simulink model "IP_nonLinearSys_Openloop_KF"  (R2015a)
settings: Solver=ode5  StartTime=0.0  StopTime=30  FixedStep=0.01  RelTol=1e-3
undefined symbols (not defined in the file): A, B, C, Continuous, D, sigbuilder_block, Time, Ts
libraries: ctrlSharedLib x1
settings Model: Creator=Fares  LastModifiedBy=Fares

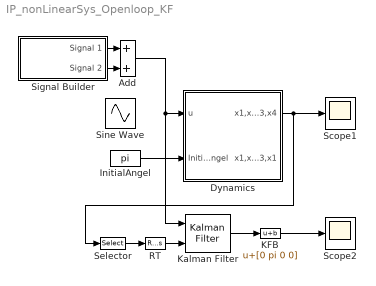
== system IP_nonLinearSys_Openloop_KF ==
  Add : Sum
  Dynamics : Subsystem  mask{mc=1.12, mpw=0.095, mps=0.025, M=9.4, fp=0.000107443, J=0.013935418, l=0.033245968, g=9.81}
      mask prompts: mc "Cart mass [kg]"; mpw "Pendulum weight mass [kg]"; mps "Pendulum stick mass [kg]"; M "Maximum control [N]"; fp "Pendulum friction [kg*m2/s]"; J "Moment of inertia [kg*m2]"; l "Distance: axis of rotation-mass center [m]"; g "Gravetational acceleration [m/s2]"
      mask init:
      | mp = mpw + mps;
      | a = l^2 + J/(mc + mp);
      | mi = (mc + mp)*l;
      mask Display: plot([0],[-2.5],[5],[4.5],[0 5],[0 0],[0 5],[0.1 0.1],[0 2],[1 1],[2.5 5],[1 1],[2 2.5 2.5 2 2],[1.25 1.25 0.75 0.75 1.25],[2.25 1.5],[1 -2.5]);
  InitialAngel : Constant  Value=pi
  KFB : Bias  Bias=[0 pi 0 0]
  Kalman Filter : ctrlSharedLib/Kalman Filter  TimeDomain=Continuous-Time  UseCurrentEstimator=on  ModelSource=Individual A, B, C, D matrices  ModelSourceVariable=ss(A,B,C,D,Ts)  A=A  B=B  C=C  D=D  NumberOfStates=1  NumberOfInputs=1  NumberOfOutputs=1  InitialEstimateSource=Dialog  X0=[0; 0; 0; 0]  P0=10  UseK=off  UseGH=off  NumberOfProcessNoiseInputs=1  G=1  TimeInvariantG=on  H=0  TimeInvariantH=on  Q=diag([1 1 500 8000])  TimeInvariantQ=on  R=diag([1e-03 0.1])  TimeInvariantR=on  N=0  TimeInvariantN=on  AddInputPort=on  AddEnablePort=off  ExternalReset=none  OutputEstimatedY=off  OutputP=off  Ts=-1
  RT : RateTransition
  Scope1 : Scope
      settings: ShowLegends=on
  Scope2 : Scope
      settings: ShowLegends=on
  Selector : Selector  InputPortWidth=4  Indices=[1 3]
  Signal Builder : Subsystem  Tag=STV Subsys  LoadFcn=sigbuilder_block('load');  StartFcn=sigbuilder_block('start');  StopFcn=sigbuilder_block('stop');  ClipboardFcn=sigbuilder_block('clipboard');  mask(Sigbuilder block){}
      mask help: Simulink:masks:SigbuilderBlock_MD
      mask init:
      | if ~strcmp(get_param(bdroot(gcbh),'SimulationStatus'),'stopped') tuvar = sigbuilder_block('maskInit'); end
      settings: CopyFcn=sigbuilder_block('copy');  DeleteFcn=sigbuilder_block('delete');  ModelCloseFcn=sigbuilder_block('modelClose');  PreSaveFcn=sigbuilder_block('preSave');  PauseFcn=sigbuilder_block('pause');  ContinueFcn=sigbuilder_block('continue');  NameChangeFcn=sigbuilder_block('namechange');  OpenFcn=sigbuilder_block('open',[437.6 199.2 550.4 400 ]);  CloseFcn=sigbuilder_block('close');
      mask Display: plot(0, 0, 100, 100,[2, 2, 32, 32, 2], [68, 8, 8, 68, 68],[32, 2], [38, 38], [32, 19, 2],[53, 60, 44], [32, 17, 17, 2],[16, 16, 31, 31]);txt = getActiveGroup(gcbh);text(2, 100, txt,'verticalAlignment', 'top');
  Sine Wave : Sin  Amplitude=0.8  SampleTime=0
  wires:
  Signal Builder/1(Signal 1) -> Add/1
  Signal Builder/2(Signal 2) -> Add/2
  InitialAngel/1 -> Dynamics/2(Initial_Angel)
  Dynamics/1(x1,x2,x3,x4) -> Selector/1, Scope1/1
  KFB/1 -> Scope2/1
  Selector/1 -> RT/1
  Kalman Filter/1 -> KFB/1
  Add/1 -> Kalman Filter/1, Dynamics/1(u)
  RT/1 -> Kalman Filter/2

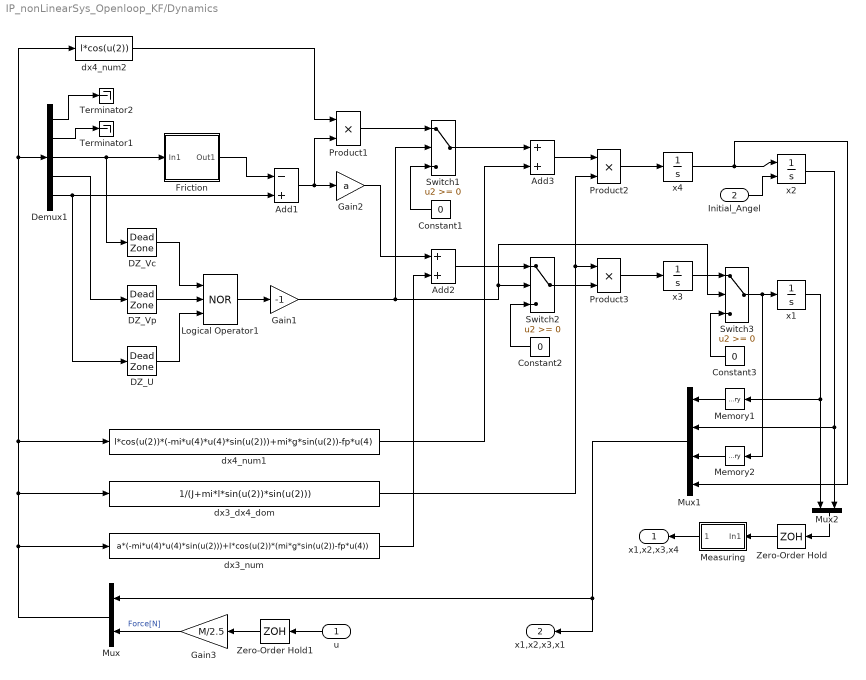
== system IP_nonLinearSys_Openloop_KF/Dynamics ==
  u : Inport
  Initial_Angel : Inport  Port=2
  " DZ_Vp" : DeadZone  LowerValue=-3.37476  UpperValue=3.37476  SaturateOnIntegerOverflow=on
  Add1 : Sum  Inputs=-+
  Add2 : Sum
  Add3 : Sum
  Constant1 : Constant  Value=0
  Constant2 : Constant  Value=0
  Constant3 : Constant  Value=0
  DZ_U : DeadZone  LowerValue=-1.37918  UpperValue=1.37918  SaturateOnIntegerOverflow=on
  DZ_Vc : DeadZone  LowerValue=-0.00793711  UpperValue=0.00793711  SaturateOnIntegerOverflow=on
  Demux1 : Demux  Outputs=5
  Friction : Subsystem  mask{FS=2.53165, FC=2.28133, DZcv=0.00793711, Xc=0.9, Yc=2.3}
      mask prompts: FS "Static friction [N]"; FC "Coulombic friction [N]"; DZcv "Minimum cart velocity [rad/s]"; Xc "Cart velocity - beginning of the linear dependence zone [m/s]"; Yc "Friction value for Xc point [N]"
      mask init:
      | small = DZcv;
      mask Display: plot([-4 4],[0 0],[-3.8 -2.4 -1.8 -1.2 -0.6 -0.2 0 0.2 0.6 1.2 1.8 2.4 3.8],[-1.4 -1 -1.1 -1.3 -1.6 -2 0 2 1.6 1.3 1.1 1 1.4]);
  Gain1 : Gain  Gain=-1
  Gain2 : Gain  Gain=a
  Gain3 : Gain  Gain=M/2.5
  Logical Operator1 : Logic  Operator=NOR  Inputs=3  AllPortsSameDT=off  OutDataTypeStr=boolean
  Measuring : Subsystem
  Memory1 : Memory
  Memory2 : Memory
  Mux : Mux  Inputs=2
  Mux1 : Mux
  Mux2 : Mux  Inputs=2
  Product1 : Product
  Product2 : Product
  Product3 : Product
  Switch1 : Switch
  Switch2 : Switch
  Switch3 : Switch
  Terminator1 : Terminator
  Terminator2 : Terminator
  Zero-Order Hold : ZeroOrderHold  SampleTime=0.01
  Zero-Order Hold1 : ZeroOrderHold  SampleTime=0.01
  dx3_dx4_dom : Fcn  Expr=1/(J+mi*l*sin(u(2))*sin(u(2)))
  dx3_num : Fcn  Expr=a*(-mi*u(4)*u(4)*sin(u(2)))+l*cos(u(2))*(mi*g*sin(u(2))-fp*u(4))
  dx4_num1 : Fcn  Expr=l*cos(u(2))*(-mi*u(4)*u(4)*sin(u(2)))+mi*g*sin(u(2))-fp*u(4)
  dx4_num2 : Fcn  Expr=l*cos(u(2))
  x1 : Integrator
  x2 : Integrator  InitialConditionSource=external  InitialCondition=pi/2
  x3 : Integrator
  x4 : Integrator
  x1,x2,x3,x4 : Outport
  x1,x2,x3,x1 : Outport  Port=2
  wires:
  DZ_U/1 -> Logical Operator1/3
  DZ_Vc/1 -> Logical Operator1/1
  Product1/1 -> Switch1/1
  Gain2/1 -> Add2/1
  Constant1/1 -> Switch1/3
  Switch2/1 -> Product3/2
  Product3/1 -> x3/1
  Logical Operator1/1 -> Gain1/1
  Constant3/1 -> Switch3/3
  Add3/1 -> Product2/1
  Demux1/1 -> Terminator2/1
  Mux/1 -> dx3_dx4_dom/1, dx4_num2/1, Demux1/1, dx4_num1/1, dx3_num/1
  dx4_num1/1 -> Add3/2
  x3/1 -> Switch3/1
  Switch3/1 -> Memory2/1, x1/1
  Add1/1 -> Gain2/1, Product1/2
  Add2/1 -> Switch2/1
  dx4_num2/1 -> Product1/1
  Demux1/3 -> Friction/1(In1), DZ_Vc/1
  Demux1/2 -> Terminator1/1
  Demux1/4 -> " DZ_Vp"/1
  Demux1/5 -> Add1/2, DZ_U/1
  " DZ_Vp"/1 -> Logical Operator1/2
  Switch1/1 -> Add3/1
  dx3_num/1 -> Add2/2
  Constant2/1 -> Switch2/3
  dx3_dx4_dom/1 -> Product2/2, Product3/1
  Product2/1 -> x4/1
  x4/1 -> x2/1, Mux1/4
  Memory2/1 -> Mux1/3
  Memory1/1 -> Mux1/1
  Mux1/1 -> x1,x2,x3,x1/1, Mux/1
  u/1 -> Zero-Order Hold1/1
  Friction/1(Out1) -> Add1/1
  Initial_Angel/1 -> x2/2
  Gain1/1 -> Switch1/2, Switch3/2, Switch2/2
  x2/1 -> Mux2/2, Mux1/2
  x1/1 -> Mux2/1, Memory1/1
  Measuring/1(Out1) -> x1,x2,x3,x4/1
  Mux2/1 -> Zero-Order Hold/1
  Zero-Order Hold/1 -> Measuring/1(In1)
  Zero-Order Hold1/1 -> Gain3/1
  Gain3/1 -> Mux/2  "Force[N]"

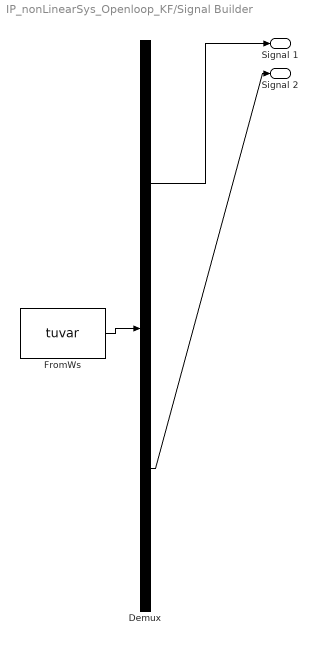
== system IP_nonLinearSys_Openloop_KF/Signal Builder ==
  Demux : Demux  Tag=STV Demux  Outputs=2
  FromWs : FromWorkspace  Tag=STV FromWs  VariableName=tuvar  SampleTime=0
      SigBuilderData=|
      | common.afterFinalStr = 'Extrapolate'
      | common.sampleTime = 0
      | dataSet.timeRange = [0 10]
      | dataSet.name = 'Group 1'
      | sbobj.Groups.Name = 'Group 1'
      | sbobj.Groups.Signals(1).Name = 'Signal 1'
      | sbobj.Groups.Signals(1).XData = [0 1 1 1.1 1.1 10]
      | sbobj.Groups.Signals(1).YData = [0 0 1.8 1.8 0 0]
      | sbobj.Groups.Signals(2).Name = 'Signal 2'
      | sbobj.Groups.Signals(2).XData = [0 5 5 5.1 5.1 10]
      | sbobj.Groups.Signals(2).YData = [0 0 -1.8 -1.8 0 0]
  Signal 1 : Outport  Tag=STV Outport
  Signal 2 : Outport  Tag=STV Outport  Port=2
  wires:
  Demux/1 -> Signal 1/1
  FromWs/1 -> Demux/1
  Demux/2 -> Signal 2/1

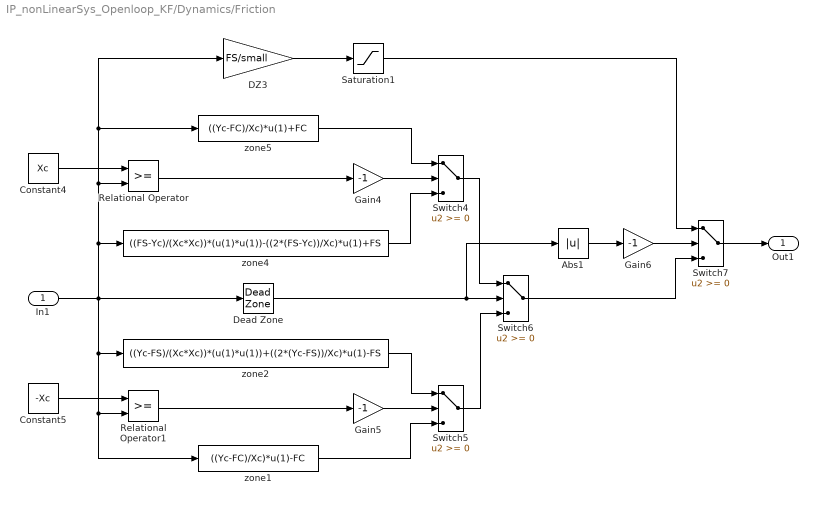
== system IP_nonLinearSys_Openloop_KF/Dynamics/Friction ==
  In1 : Inport
  Abs1 : Abs
  Constant4 : Constant  Value=Xc
  Constant5 : Constant  Value=-Xc
  DZ3 : Gain  Gain=FS/small
  Dead Zone : DeadZone  LowerValue=-DZcv  UpperValue=DZcv  SaturateOnIntegerOverflow=on
  Gain4 : Gain  Gain=-1
  Gain5 : Gain  Gain=-1
  Gain6 : Gain  Gain=-1
  Relational Operator : RelationalOperator  OutDataTypeStr=boolean
  Relational Operator1 : RelationalOperator  OutDataTypeStr=boolean
  Saturation1 : Saturate  UpperLimit=FS  LowerLimit=-FS
  Switch{4..7} (4 alike) : Switch
  zone1 : Fcn  Expr=((Yc-FC)/Xc)*u(1)-FC
  zone2 : Fcn  Expr=((Yc-FS)/(Xc*Xc))*(u(1)*u(1))+((2*(Yc-FS))/Xc)*u(1)-FS
  zone4 : Fcn  Expr=((FS-Yc)/(Xc*Xc))*(u(1)*u(1))-((2*(FS-Yc))/Xc)*u(1)+FS
  zone5 : Fcn  Expr=((Yc-FC)/Xc)*u(1)+FC
  Out1 : Outport
  wires:
  Gain4/1 -> Switch4/2
  Dead Zone/1 -> Abs1/1, Switch6/2
  Gain5/1 -> Switch5/2
  Relational Operator/1 -> Gain4/1
  Constant5/1 -> Relational Operator1/1
  Relational Operator1/1 -> Gain5/1
  Abs1/1 -> Gain6/1
  DZ3/1 -> Saturation1/1
  Switch6/1 -> Switch7/3
  Switch4/1 -> Switch6/1
  zone2/1 -> Switch5/1
  Gain6/1 -> Switch7/2
  zone4/1 -> Switch4/3
  Switch7/1 -> Out1/1
  In1/1 -> zone1/1, Relational Operator1/2, zone2/1, DZ3/1, zone5/1, Relational Operator/2, zone4/1, Dead Zone/1
  Saturation1/1 -> Switch7/1
  zone5/1 -> Switch4/1
  Constant4/1 -> Relational Operator/1
  zone1/1 -> Switch5/3
  Switch5/1 -> Switch6/3

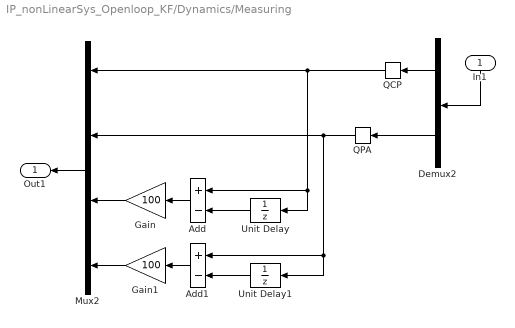
== system IP_nonLinearSys_Openloop_KF/Dynamics/Measuring ==
  In1 : Inport
  Add : Sum  Inputs=+-
  Add1 : Sum  Inputs=+-
  Demux2 : Demux  Outputs=2
  Gain : Gain  Gain=100
  Gain1 : Gain  Gain=100
  Mux2 : Mux
  QCP : Quantizer  QuantizationInterval=0.156/2048
  QPA : Quantizer  QuantizationInterval=(2*pi)/2048
  Unit Delay : UnitDelay  SampleTime=-1
  Unit Delay1 : UnitDelay  SampleTime=-1
  Out1 : Outport
  wires:
  Demux2/1 -> QCP/1
  Mux2/1 -> Out1/1
  In1/1 -> Demux2/1
  QPA/1 -> Unit Delay1/1, Add1/1, Mux2/2
  QCP/1 -> Unit Delay/1, Add/1, Mux2/1
  Demux2/2 -> QPA/1
  Unit Delay1/1 -> Add1/2
  Unit Delay/1 -> Add/2
  Add1/1 -> Gain1/1
  Add/1 -> Gain/1
  Gain1/1 -> Mux2/4
  Gain/1 -> Mux2/3
